simulink model "w_f"  (R2024a)
settings: Solver=VariableStepAuto  StartTime=0.0  StopTime=10.0  RelTol=1e-3
values from neighbouring files (symbols this model uses):
  A = [8 1 11; 4 0 4; -4 -3 -7]    [init.m]
  B = [-1; -3; 3]    [init.m]
  B_f = [1, -1 ... (first row only)    [init.m]
  C = [-2 0 -3]    [init.m]
  D = 15    [init.m]
  D_f = [0, 3]    [init.m]
  Gamma_f = [35, 10, -28, 17 ... (first row only)    [init.m]
  Gamma_g = [0 0 0 ... (first row only)    [init.m]
  K = [-3.5, 1, -3.5]    [init.m]
  K_f = [-2.6629 , -0.9070 , 2.2585 , -1.3262]    [init.m]    (also in tester.m = [real(Kf_complex(1)), imag(Kf_complex(1)), real(Kf_complex(3)
  K_g = [-0.7552 , -0.1012 , 1.4675]    [init.m]    (also in tester.m = [real(Kg0), real(Kg2), imag(Kg2)])
  wf0 = [1; 1; 1; 1]    [init.m]
  wg0 = [1; -1; 0]    [init.m]
  x0 = [0; 0; 0]    [init.m]
  Y_f = [-6, -2, 4, -3 ... (first row only)    [init.m]
  Y_g = [-12, 0, 21]    [init.m]
settings Model: Creator=eva  LastModifiedBy=eva

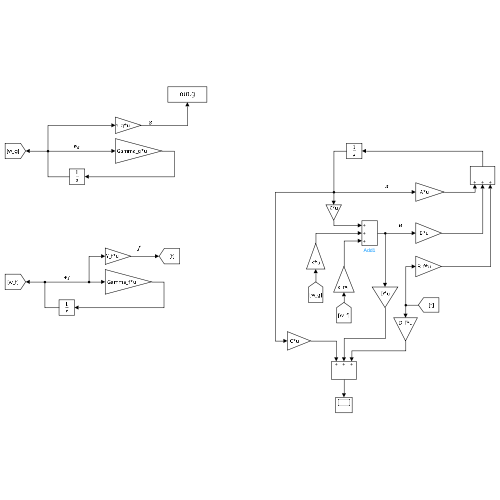
[thumbnail: Simulink's stored preview of the top-level diagram]
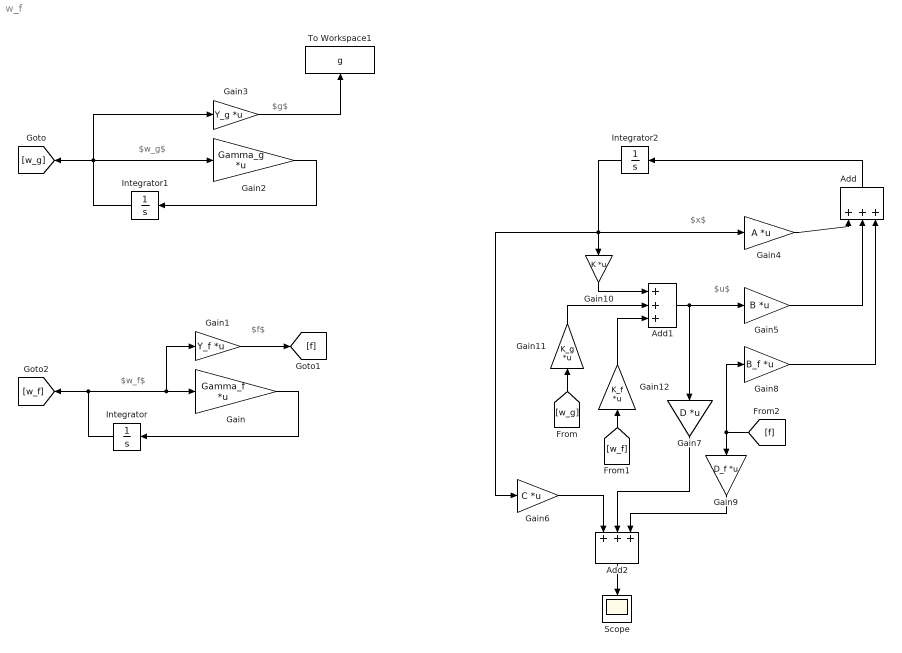
== system w_f ==
  note: $x$
  note: $w_f$
  note: $f$
  note: $w_g$
  note: $g$
  note: $u$
  Add : Sum  Inputs=+++
  Add1 : Sum  Inputs=+++
  Add2 : Sum  Inputs=+++
  Gain : Gain  Gain=Gamma_f  Multiplication=Matrix(K*u)
  Gain1 : Gain  Gain=Y_f  Multiplication=Matrix(K*u)
  Gain10 : Gain  Gain=K  Multiplication=Matrix(K*u)
  Gain11 : Gain  Gain=K_g  Multiplication=Matrix(K*u)
  Gain12 : Gain  Gain=K_f  Multiplication=Matrix(K*u)
  Gain2 : Gain  Gain=Gamma_g  Multiplication=Matrix(K*u)
  Gain3 : Gain  Gain=Y_g  Multiplication=Matrix(K*u)
  Gain4 : Gain  Gain=A  Multiplication=Matrix(K*u)
  Gain5 : Gain  Gain=B  Multiplication=Matrix(K*u)
  Gain6 : Gain  Gain=C  Multiplication=Matrix(K*u)
  Gain7 : Gain  Gain=D  Multiplication=Matrix(K*u)
  Gain8 : Gain  Gain=B_f  Multiplication=Matrix(K*u)
  Gain9 : Gain  Gain=D_f  Multiplication=Matrix(K*u)
  Integrator : Integrator  InitialCondition=wf0
  Integrator1 : Integrator  InitialCondition=wg0
  Integrator2 : Integrator  InitialCondition=x0
  Scope : Scope
  To Workspace1 : ToWorkspace  VariableName=g  SaveFormat=Structure With Time  SampleTime=-1
  wires:
  Integrator/1 -> Gain1/1, Gain/1, [w_f]
  Gain/1 -> Integrator/1
  Gain2/1 -> Integrator1/1
  Gain3/1 -> To Workspace1/1
  Integrator1/1 -> Gain3/1, [w_g], Gain2/1
  Integrator2/1 -> Gain10/1, Gain6/1, Gain4/1
  Gain4/1 -> Add/1
  Gain5/1 -> Add/2
  Add/1 -> Integrator2/1
  Add1/1 -> Gain5/1, Gain7/1
  Gain10/1 -> Add1/1
  Gain11/1 -> Add1/2
  Gain12/1 -> Add1/3
  Gain8/1 -> Add/3
  Add2/1 -> Scope/1
  [w_g] -> Gain11/1
  Gain1/1 -> [f]
  [w_f] -> Gain12/1
  [f] -> Gain8/1, Gain9/1
  Gain9/1 -> Add2/3
  Gain7/1 -> Add2/2
  Gain6/1 -> Add2/1
